simulink model "motor"  (R2020b)
settings: Solver=VariableStepAuto  StartTime=0.0  StopTime=10.0  RelTol=1e-3
values from neighbouring files (symbols this model uses):
  J = 6.04e-06    [variables_values.mat]
  Lam = 0.0165    [variables_values.mat]
  Lss = 0.0101    [variables_values.mat]
  rs = 5.2    [variables_values.mat]
  Ts = 0.001942    [variables_values.mat]
undefined symbols (not defined in the file or in its folder): Dm, P
settings Model: Creator=omkar  LastModifiedBy=DELL

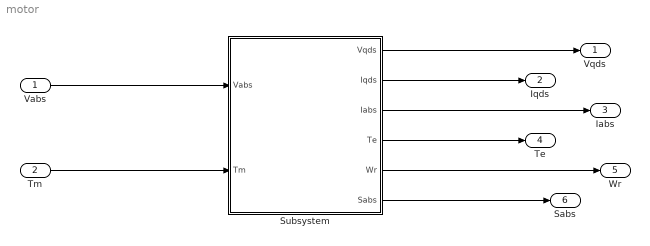
== system motor ==
  Vabs : Inport
  Tm : Inport  Port=2
  Subsystem : Subsystem
  Vqds : Outport
  Iqds : Outport  Port=2
  Iabs : Outport  Port=3
  Te : Outport  Port=4
  Wr : Outport  Port=5
  Sabs : Outport  Port=6
  wires:
  Vabs/1 -> Subsystem/1(Vabs)
  Tm/1 -> Subsystem/2(Tm)
  Subsystem/1(Vqds) -> Vqds/1
  Subsystem/2(Iqds) -> Iqds/1
  Subsystem/3(Iabs) -> Iabs/1
  Subsystem/4(Te) -> Te/1
  Subsystem/5(Wr) -> Wr/1
  Subsystem/6(Sabs) -> Sabs/1

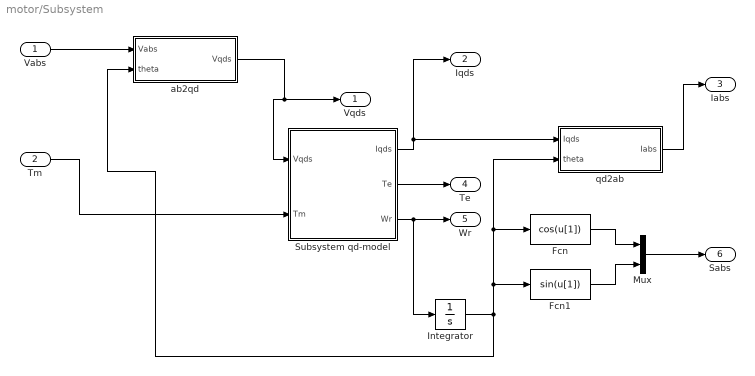
== system motor/Subsystem ==
  Vabs : Inport
  Tm : Inport  Port=2
  Fcn : Fcn  Expr=cos(u[1])
  Fcn1 : Fcn
  Integrator : Integrator
  Mux : Mux  Inputs=2
  Subsystem qd-model : Subsystem
  ab2qd : Subsystem
  qd2ab : Subsystem
  Vqds : Outport
  Iqds : Outport  Port=2
  Iabs : Outport  Port=3
  Te : Outport  Port=4
  Wr : Outport  Port=5
  Sabs : Outport  Port=6
  wires:
  Subsystem qd-model/2(Te) -> Te/1
  Fcn/1 -> Mux/1
  qd2ab/1(" Iabs") -> Iabs/1
  Integrator/1 -> ab2qd/2(theta), Fcn1/1, qd2ab/2(theta), Fcn/1
  ab2qd/1(" Vqds") -> Vqds/1, Subsystem qd-model/1(Vqds)
  Subsystem qd-model/1(Iqds) -> Iqds/1, qd2ab/1(Iqds)
  Subsystem qd-model/3(Wr) -> Wr/1, Integrator/1
  Fcn1/1 -> Mux/2
  Vabs/1 -> ab2qd/1(Vabs)
  Tm/1 -> Subsystem qd-model/2(Tm)
  Mux/1 -> Sabs/1

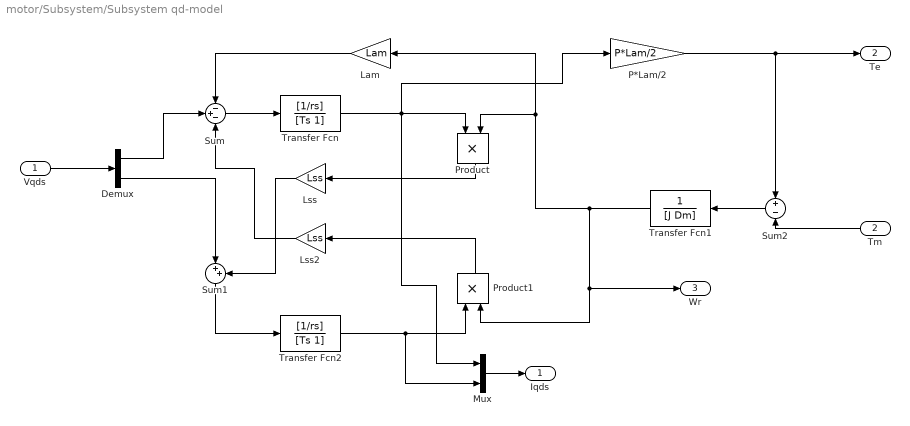
== system motor/Subsystem/Subsystem qd-model ==
  Vqds : Inport
  Tm : Inport  Port=2
  Demux : Demux  Outputs=2
  Lam : Gain  Gain=Lam
  Lss : Gain  Gain=Lss
  Lss2 : Gain  Gain=Lss
  Mux : Mux  Inputs=2
  P*Lam/2 : Gain  Gain=P*Lam/2
  Product : Product
  Product1 : Product
  Sum : Sum  Inputs=-+-
  Sum1 : Sum  Inputs=|++
  Sum2 : Sum  Inputs=+-
  Transfer Fcn : TransferFcn  Numerator=[1/rs]  Denominator=[Ts 1]
  Transfer Fcn1 : TransferFcn  Denominator=[J Dm]
  Transfer Fcn2 : TransferFcn  Numerator=[1/rs]  Denominator=[Ts 1]
  Iqds : Outport
  Te : Outport  Port=2
  Wr : Outport  Port=3
  wires:
  Vqds/1 -> Demux/1
  Demux/1 -> Sum/2
  Demux/2 -> Sum1/1
  P*Lam/2/1 -> Sum2/1, Te/1
  Tm/1 -> Sum2/2
  Sum/1 -> Transfer Fcn/1
  Lam/1 -> Sum/1
  Lss2/1 -> Sum/3
  Lss/1 -> Sum1/2
  Sum1/1 -> Transfer Fcn2/1
  Sum2/1 -> Transfer Fcn1/1
  Transfer Fcn2/1 -> Mux/2, Product1/1
  Product1/1 -> Lss2/1
  Product/1 -> Lss/1
  Transfer Fcn/1 -> Mux/1, P*Lam/2/1, Product/1
  Transfer Fcn1/1 -> Product/2, Lam/1, Product1/2, Wr/1
  Mux/1 -> Iqds/1

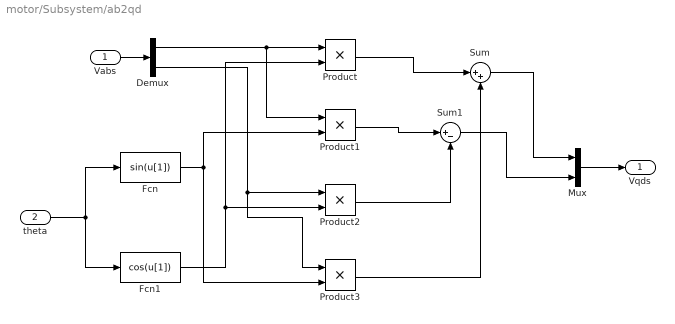
== system motor/Subsystem/ab2qd ==
  Vabs : Inport
  theta : Inport  Port=2
  Demux : Demux  Outputs=2
  Fcn : Fcn
  Fcn1 : Fcn  Expr=cos(u[1])
  Mux : Mux  Inputs=2
  Product{,1..3} (4 alike) : Product
  Sum : Sum  Inputs=|++
  Sum1 : Sum  Inputs=|+-
  " Vqds" : Outport
  wires:
  Vabs/1 -> Demux/1
  Mux/1 -> " Vqds"/1
  theta/1 -> Fcn/1, Fcn1/1
  Demux/1 -> Product1/1, Product/1
  Fcn1/1 -> Product2/2, Product/2
  Fcn/1 -> Product1/2, Product3/2
  Demux/2 -> Product3/1, Product2/1
  Product/1 -> Sum/1
  Product3/1 -> Sum/2
  Sum/1 -> Mux/1
  Product1/1 -> Sum1/1
  Product2/1 -> Sum1/2
  Sum1/1 -> Mux/2

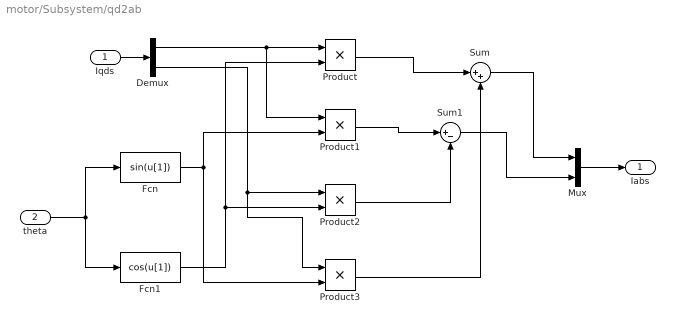
== system motor/Subsystem/qd2ab ==
  Iqds : Inport
  theta : Inport  Port=2
  Demux : Demux  Outputs=2
  Fcn : Fcn
  Fcn1 : Fcn  Expr=cos(u[1])
  Mux : Mux  Inputs=2
  Product{,1..3} (4 alike) : Product
  Sum : Sum  Inputs=|++
  Sum1 : Sum  Inputs=|+-
  " Iabs" : Outport
  wires:
  Iqds/1 -> Demux/1
  Mux/1 -> " Iabs"/1
  theta/1 -> Fcn/1, Fcn1/1
  Demux/1 -> Product1/1, Product/1
  Fcn1/1 -> Product2/2, Product/2
  Fcn/1 -> Product1/2, Product3/2
  Demux/2 -> Product3/1, Product2/1
  Product/1 -> Sum/1
  Product3/1 -> Sum/2
  Sum/1 -> Mux/1
  Product1/1 -> Sum1/1
  Product2/1 -> Sum1/2
  Sum1/1 -> Mux/2
